simulink model "drone_model"  (R2020b)
settings: Solver=FixedStepAuto  StartTime=0.0  StopTime=30  FixedStep=0.01  RelTol=1e-3
undefined symbols (not defined in the file or in its folder): cd, clientID, d, g, I, Kf, Km, m, rho, sendCoppelia, sim
libraries: pid_lib x6, vrlib x1
settings Model: Creator=roger  LastModifiedBy=Guillermo
settings DataIOCC: ReturnWorkspaceOutputs=off

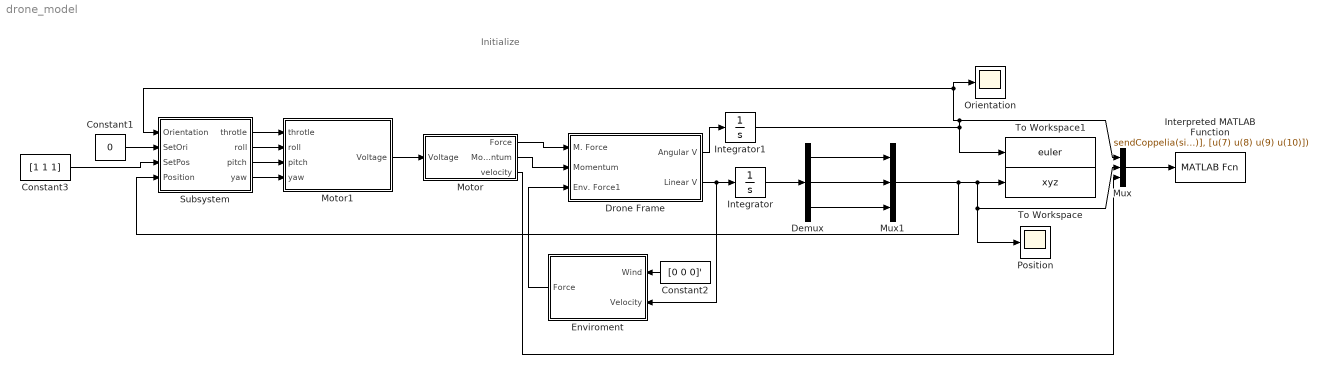
== system drone_model ==
  note: Initialize
  Constant1 : Constant  Value=0
  Constant2 : Constant  Value=[0 0 0]'  VectorParams1D=off
  Constant3 : Constant  Value=[1 1 1]
  Demux : Demux  Outputs=3
  Drone Frame : Subsystem
  Enviroment : Subsystem
  Integrator : Integrator
  Integrator1 : Integrator
  Interpreted MATLAB Function : MATLABFcn  MATLABFcn=sendCoppelia(sim, clientID, [u(4) u(5) u(6)], [u(1) u(2) u(3)], [u(7) u(8) u(9) u(10)])  OutputDimensions=0
  Motor : Subsystem
  Motor1 : Subsystem
  Mux : Mux  Inputs=3
  Mux1 : Mux  Inputs=3
  Orientation : Scope
  Position : Scope
  Subsystem : Subsystem
  To Workspace : ToWorkspace  VariableName=xyz  SaveFormat=Timeseries  SampleTime=-1
  To Workspace1 : ToWorkspace  VariableName=euler  SaveFormat=Timeseries  SampleTime=-1
  wires:
  Drone Frame/2(Linear V) -> Enviroment/2(Velocity), Integrator/1
  Drone Frame/1(Angular V) -> Integrator1/1
  Integrator1/1 -> To Workspace1/1, Mux/1, Subsystem/1(Orientation), Orientation/1
  Motor/1(Force) -> Drone Frame/1(M. Force)
  Motor/2(Momentum) -> Drone Frame/2(Momentum)
  Enviroment/1(Force) -> Drone Frame/3(Env. Force1)
  Constant2/1 -> Enviroment/1(Wind)
  Motor1/1(Voltage) -> Motor/1(Voltage)
  Integrator/1 -> Demux/1
  Subsystem/1(throtle) -> Motor1/1(throtle)
  Subsystem/2(roll) -> Motor1/2(roll)
  Subsystem/3(pitch) -> Motor1/3(pitch)
  Constant3/1 -> Subsystem/3(SetPos)
  Constant1/1 -> Subsystem/2(SetOri)
  Mux/1 -> Interpreted MATLAB Function/1
  Subsystem/4(yaw) -> Motor1/4(yaw)
  Mux1/1 -> Subsystem/4(Position), To Workspace/1, Mux/2, Position/1
  Demux/1 -> Mux1/1
  Demux/2 -> Mux1/2
  Demux/3 -> Mux1/3
  Motor/3(velocity) -> Mux/3

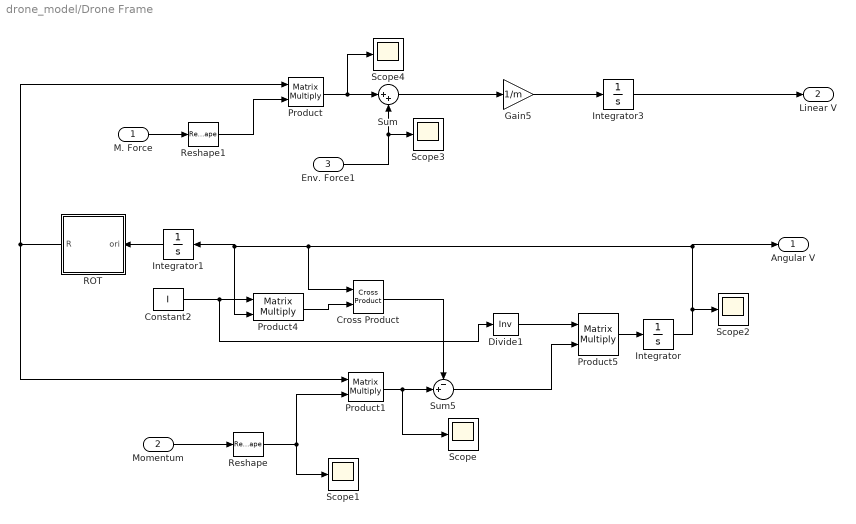
== system drone_model/Drone Frame ==
  M. Force : Inport
  Momentum : Inport  Port=2
  Env. Force1 : Inport  Port=3
  Constant2 : Constant  Value=I
  Cross Product : vrlib/Utilities/Cross Product
  Divide1 : Product  Inputs=/  Multiplication=Matrix(*)
  Gain5 : Gain  Gain=1/m
  Integrator : Integrator
  Integrator1 : Integrator
  Integrator3 : Integrator
  Product{,1,4..5} (4 alike) : Product  Multiplication=Matrix(*)
  ROT : MATLAB Function  TreatAsAtomicUnit=on
  Reshape : Reshape  OutputDimensionality=Column vector (2-D)
  Reshape1 : Reshape  OutputDimensionality=Column vector (2-D)
  Scope{,1..4} (5 alike) : Scope
  Sum : Sum  Inputs=|++
  Sum5 : Sum  Inputs=-+|
  Angular V : Outport
  Linear V : Outport  Port=2
  wires:
  Product/1 -> Scope4/1, Sum/1
  Sum5/1 -> Product5/2
  Gain5/1 -> Integrator3/1
  Sum/1 -> Gain5/1
  Product5/1 -> Integrator/1
  Integrator/1 -> Scope2/1, Integrator1/1, Product4/2, Cross Product/1, Angular V/1
  Cross Product/1 -> Sum5/1
  Divide1/1 -> Product5/1
  Constant2/1 -> Divide1/1, Product4/1
  Product4/1 -> Cross Product/2
  Integrator3/1 -> Linear V/1
  Momentum/1 -> Reshape/1
  M. Force/1 -> Reshape1/1
  Reshape1/1 -> Product/2
  Reshape/1 -> Scope1/1, Product1/2
  Product1/1 -> Scope/1, Sum5/2
  Env. Force1/1 -> Scope3/1, Sum/2
  Integrator1/1 -> ROT/1(ori)
  ROT/1(R) -> Product1/1, Product/1

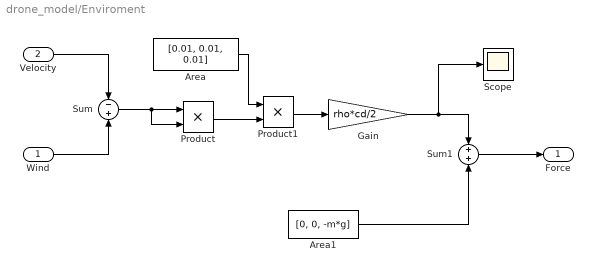
== system drone_model/Enviroment ==
  Wind : Inport
  Velocity : Inport  Port=2
  Area : Constant  Value=[0.01, 0.01, 0.01]
  Area1 : Constant  Value=[0, 0, -m*g]
  Gain : Gain  Gain=rho*cd/2
  Product : Product
  Product1 : Product
  Scope : Scope
  Sum : Sum  Inputs=-|+
  Sum1 : Sum  Inputs=+|+
  Force : Outport
  wires:
  Wind/1 -> Sum/2
  Velocity/1 -> Sum/1
  Sum/1 -> Product/2, Product/1
  Product/1 -> Product1/2
  Area/1 -> Product1/1
  Sum1/1 -> Force/1
  Area1/1 -> Sum1/2
  Product1/1 -> Gain/1
  Gain/1 -> Scope/1, Sum1/1

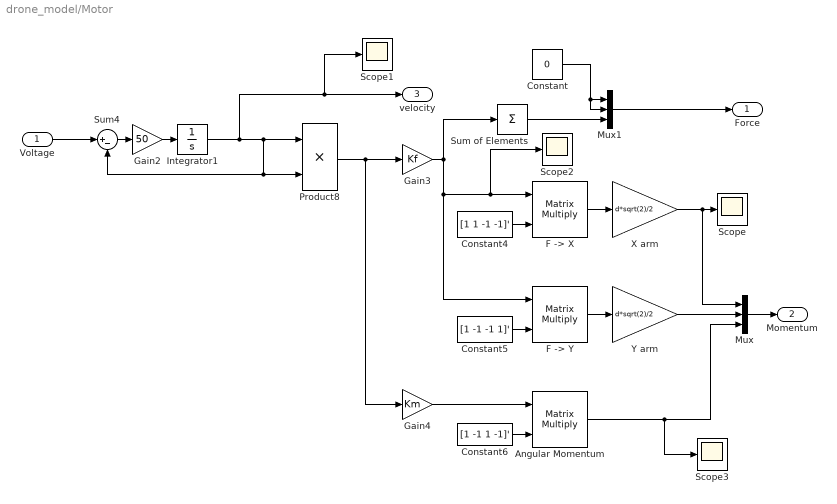
== system drone_model/Motor ==
  Voltage : Inport
  Angular Momentum : Product  Multiplication=Matrix(*)
  Constant : Constant  Value=0
  Constant4 : Constant  Value=[1 1 -1 -1]'  VectorParams1D=off
  Constant5 : Constant  Value=[1 -1 -1 1]'  VectorParams1D=off
  Constant6 : Constant  Value=[1 -1 1 -1]'  VectorParams1D=off
  "F -> X" : Product  Multiplication=Matrix(*)
  "F -> Y" : Product  Multiplication=Matrix(*)
  Gain2 : Gain  Gain=50
  Gain3 : Gain  Gain=Kf
  Gain4 : Gain  Gain=Km
  Integrator1 : Integrator
  Mux : Mux  Inputs=3
  Mux1 : Mux  Inputs=3
  Product8 : Product
  Scope{,1..3} (4 alike) : Scope
  Sum of Elements : Sum  Inputs=+
  Sum4 : Sum  Inputs=|+-
  X arm : Gain  Gain=d*sqrt(2)/2
  Y arm : Gain  Gain=d*sqrt(2)/2
  Force : Outport
  Momentum : Outport  Port=2
  velocity : Outport  Port=3
  wires:
  Gain3/1 -> Scope2/1, "F -> X"/1, "F -> Y"/1, Sum of Elements/1
  Sum4/1 -> Gain2/1
  Gain4/1 -> Angular Momentum/1
  Product8/1 -> Gain3/1, Gain4/1
  Integrator1/1 -> Scope1/1, velocity/1, Product8/1, Product8/2, Sum4/2
  "F -> Y"/1 -> Y arm/1
  Gain2/1 -> Integrator1/1
  Constant4/1 -> "F -> X"/2
  Constant6/1 -> Angular Momentum/2
  Constant5/1 -> "F -> Y"/2
  Voltage/1 -> Sum4/1
  "F -> X"/1 -> X arm/1
  X arm/1 -> Scope/1, Mux/1
  Y arm/1 -> Mux/2
  Angular Momentum/1 -> Scope3/1, Mux/3
  Mux/1 -> Momentum/1
  Sum of Elements/1 -> Mux1/3
  Mux1/1 -> Force/1
  Constant/1 -> Mux1/2, Mux1/1

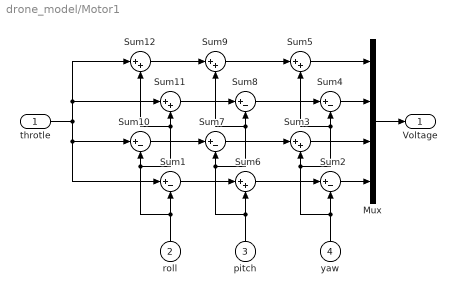
== system drone_model/Motor1 ==
  throtle : Inport
  roll : Inport  Port=2
  pitch : Inport  Port=3
  yaw : Inport  Port=4
  Mux : Mux
  Sum{1..2,4,7..8,10} (6 alike) : Sum  Inputs=|+-
  Sum{3,5..6,9,11..12} (6 alike) : Sum  Inputs=|++
  Voltage : Outport
  wires:
  Mux/1 -> Voltage/1
  Sum2/1 -> Mux/4
  yaw/1 -> Sum3/2, Sum5/2, Sum4/2, Sum2/2
  Sum3/1 -> Mux/3
  Sum4/1 -> Mux/2
  Sum5/1 -> Mux/1
  Sum8/1 -> Sum4/1
  Sum6/1 -> Sum2/1
  Sum9/1 -> Sum5/1
  Sum7/1 -> Sum3/1
  pitch/1 -> Sum7/2, Sum9/2, Sum8/2, Sum6/2
  throtle/1 -> Sum10/1, Sum1/1, Sum12/1, Sum11/1
  Sum11/1 -> Sum8/1
  Sum1/1 -> Sum6/1
  Sum12/1 -> Sum9/1
  Sum10/1 -> Sum7/1
  roll/1 -> Sum10/2, Sum12/2, Sum11/2, Sum1/2

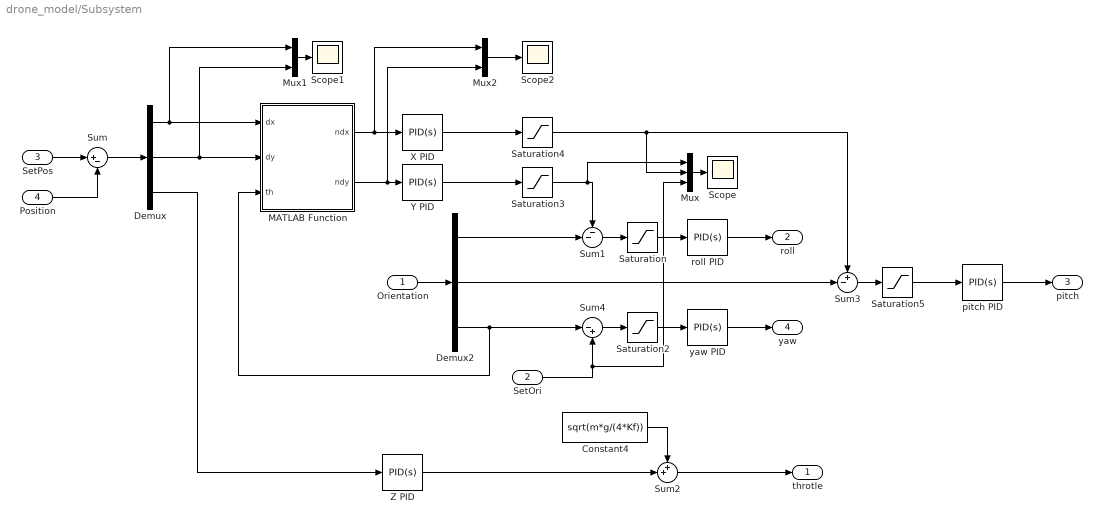
== system drone_model/Subsystem ==
  Orientation : Inport
  SetOri : Inport  Port=2
  SetPos : Inport  Port=3
  Position : Inport  Port=4
  Constant4 : Constant  Value=sqrt(m*g/(4*Kf))
  Demux : Demux  Outputs=3
  Demux2 : Demux  Outputs=3
  MATLAB Function : MATLAB Function  TreatAsAtomicUnit=on
  Mux : Mux  Inputs=3
  Mux1 : Mux  Inputs=2
  Mux2 : Mux  Inputs=2
  Saturation : Saturate  UpperLimit=0.01  LowerLimit=-0.01
  Saturation2 : Saturate  UpperLimit=0.01  LowerLimit=-0.01
  Saturation3 : Saturate  UpperLimit=0.05  LowerLimit=-0.05
  Saturation4 : Saturate  UpperLimit=0.05  LowerLimit=-0.05
  Saturation5 : Saturate  UpperLimit=0.01  LowerLimit=-0.01
  Scope : Scope
  Scope1 : Scope
  Scope2 : Scope
  Sum : Sum  Inputs=|+-
  Sum1 : Sum  Inputs=--|
  Sum2 : Sum  Inputs=++|
  Sum3 : Sum  Inputs=+-|
  Sum4 : Sum  Inputs=|-+
  X PID : pid_lib/PID Controller  Controller=PID  Form=Parallel  TimeDomain=Continuous-time  UseExternalTs=off  SampleTime=-1  IntegratorMethod=Forward Euler  FilterMethod=Forward Euler  ControllerParametersSource=internal  P=0.1  I=0  D=0.2  UseFilter=on  N=100  TunerSelectOption=Transfer Function Based (PID Tuner App)  InitialConditionSource=internal  InitialConditionForIntegrator=0  InitialConditionForFilter=0  DifferentiatorICPrevScaledInput=0  ExternalReset=none  TrackingMode=off  Kt=1  LimitOutput=off  SatLimitsSource=internal  UpperSaturationLimit=inf  LowerSaturationLimit=-inf  LinearizeAsGain=on  AntiWindupMode=none  Kb=1  POutMin=[]  POutMax=[]  IOutMin=[]  IOutMax=[]  DOutMin=[]  DOutMax=[]  NOutMin=[]  NOutMax=[]  SumOutMin=[]  SumOutMax=[]  SaturationOutMin=[]  SaturationOutMax=[]  PParamMin=[]  PParamMax=[]  IParamMin=[]  IParamMax=[]  DParamMin=[]  DParamMax=[]  NParamMin=[]  NParamMax=[]  KbParamMin=[]  KbParamMax=[]  KtParamMin=[]  KtParamMax=[]  KbOutMin=[]  KbOutMax=[]  KtOutMin=[]  KtOutMax=[]  IntegratorOutMin=[]  IntegratorOutMax=[]  FilterOutMin=[]  FilterOutMax=[]  SumI1OutMin=[]  SumI1OutMax=[]  SumI2OutMin=[]  SumI2OutMax=[]  SumI3OutMin=[]  SumI3OutMax=[]  SumI4OutMin=[]  SumI4OutMax=[]  SumDOutMin=[]  SumDOutMax=[]  DifferentiatorOutMin=[]  DifferentiatorOutMax=[]  FilterDiffOutCoefMin=[]  FilterDiffOutCoefMax=[]  ReciprocalOutMin=[]  ReciprocalOutMax=[]  SumDenOutMin=[]  SumDenOutMax=[]  SumNumOutMin=[]  SumNumOutMax=[]  DivideOutMin=[]  DivideOutMax=[]  UdiffTsProdOutMin=[]  UdiffTsProdOutMax=[]  NTsProdOutMin=[]  NTsProdOutMax=[]  UintegralTsProdOutMin=[]  UintegralTsProdOutMax=[]  UngainTsProdOutMin=[]  UngainTsProdOutMax=[]  IntegratorContinuousStateAttributes=''  IntegratorStateMustResolveToSignalObject=off  IntegratorRTWStateStorageClass=Auto  FilterContinuousStateAttributes=''  FilterStateMustResolveToSignalObject=off  FilterRTWStateStorageClass=Auto  ParallelPVariant=InternalParameters  IdealPVariant=Disabled  IVariant=InternalParameters  DVariant=InternalParameters  IntegratorVariant=Continuous  SatVariant=Disabled  AWVariant=Passthrough  PCopyVariant=Disabled  TRVariant=Disabled  FdbkBlocksVariant=Forward  IdealPFdbkVariant=Disabled  SatFdbkVariant=Disabled  DerivativeFilterVariant=ContFilter  NVariant=InternalParameters  NCopyVariant=Disabled  FilterICVariant=InternalICsFilter  IntegratorICVariant=InternalICs  ExternalResetVariant=Disabled  TRSumVariant=Passthrough  SumFdbkVariant=Disabled  SumVariant=Sum_PID  TsampFilterVariant=InternalTs  TsampNgainVariant=Passthrough  TsampIntegralVariant=Passthrough  ExternalSaturationOutDataTypeStr=Inherit: Same as second input
  Y PID : pid_lib/PID Controller  Controller=PID  Form=Parallel  TimeDomain=Continuous-time  UseExternalTs=off  SampleTime=-1  IntegratorMethod=Forward Euler  FilterMethod=Forward Euler  ControllerParametersSource=internal  P=0.1  I=0  D=0.2  UseFilter=on  N=100  TunerSelectOption=Transfer Function Based (PID Tuner App)  InitialConditionSource=internal  InitialConditionForIntegrator=0  InitialConditionForFilter=0  DifferentiatorICPrevScaledInput=0  ExternalReset=none  TrackingMode=off  Kt=1  LimitOutput=off  SatLimitsSource=internal  UpperSaturationLimit=inf  LowerSaturationLimit=-inf  LinearizeAsGain=on  AntiWindupMode=none  Kb=1  POutMin=[]  POutMax=[]  IOutMin=[]  IOutMax=[]  DOutMin=[]  DOutMax=[]  NOutMin=[]  NOutMax=[]  SumOutMin=[]  SumOutMax=[]  SaturationOutMin=[]  SaturationOutMax=[]  PParamMin=[]  PParamMax=[]  IParamMin=[]  IParamMax=[]  DParamMin=[]  DParamMax=[]  NParamMin=[]  NParamMax=[]  KbParamMin=[]  KbParamMax=[]  KtParamMin=[]  KtParamMax=[]  KbOutMin=[]  KbOutMax=[]  KtOutMin=[]  KtOutMax=[]  IntegratorOutMin=[]  IntegratorOutMax=[]  FilterOutMin=[]  FilterOutMax=[]  SumI1OutMin=[]  SumI1OutMax=[]  SumI2OutMin=[]  SumI2OutMax=[]  SumI3OutMin=[]  SumI3OutMax=[]  SumI4OutMin=[]  SumI4OutMax=[]  SumDOutMin=[]  SumDOutMax=[]  DifferentiatorOutMin=[]  DifferentiatorOutMax=[]  FilterDiffOutCoefMin=[]  FilterDiffOutCoefMax=[]  ReciprocalOutMin=[]  ReciprocalOutMax=[]  SumDenOutMin=[]  SumDenOutMax=[]  SumNumOutMin=[]  SumNumOutMax=[]  DivideOutMin=[]  DivideOutMax=[]  UdiffTsProdOutMin=[]  UdiffTsProdOutMax=[]  NTsProdOutMin=[]  NTsProdOutMax=[]  UintegralTsProdOutMin=[]  UintegralTsProdOutMax=[]  UngainTsProdOutMin=[]  UngainTsProdOutMax=[]  IntegratorContinuousStateAttributes=''  IntegratorStateMustResolveToSignalObject=off  IntegratorRTWStateStorageClass=Auto  FilterContinuousStateAttributes=''  FilterStateMustResolveToSignalObject=off  FilterRTWStateStorageClass=Auto  ParallelPVariant=InternalParameters  IdealPVariant=Disabled  IVariant=InternalParameters  DVariant=InternalParameters  IntegratorVariant=Continuous  SatVariant=Disabled  AWVariant=Passthrough  PCopyVariant=Disabled  TRVariant=Disabled  FdbkBlocksVariant=Forward  IdealPFdbkVariant=Disabled  SatFdbkVariant=Disabled  DerivativeFilterVariant=ContFilter  NVariant=InternalParameters  NCopyVariant=Disabled  FilterICVariant=InternalICsFilter  IntegratorICVariant=InternalICs  ExternalResetVariant=Disabled  TRSumVariant=Passthrough  SumFdbkVariant=Disabled  SumVariant=Sum_PID  TsampFilterVariant=InternalTs  TsampNgainVariant=Passthrough  TsampIntegralVariant=Passthrough  ExternalSaturationOutDataTypeStr=Inherit: Same as second input
  Z PID : pid_lib/PID Controller  Controller=PID  Form=Parallel  TimeDomain=Continuous-time  UseExternalTs=off  SampleTime=-1  IntegratorMethod=Forward Euler  FilterMethod=Forward Euler  ControllerParametersSource=internal  P=0.05  I=0  D=0.2  UseFilter=on  N=100  TunerSelectOption=Transfer Function Based (PID Tuner App)  InitialConditionSource=internal  InitialConditionForIntegrator=0  InitialConditionForFilter=0  DifferentiatorICPrevScaledInput=0  ExternalReset=none  TrackingMode=off  Kt=1  LimitOutput=off  SatLimitsSource=internal  UpperSaturationLimit=inf  LowerSaturationLimit=-inf  LinearizeAsGain=on  AntiWindupMode=none  Kb=1  POutMin=[]  POutMax=[]  IOutMin=[]  IOutMax=[]  DOutMin=[]  DOutMax=[]  NOutMin=[]  NOutMax=[]  SumOutMin=[]  SumOutMax=[]  SaturationOutMin=[]  SaturationOutMax=[]  PParamMin=[]  PParamMax=[]  IParamMin=[]  IParamMax=[]  DParamMin=[]  DParamMax=[]  NParamMin=[]  NParamMax=[]  KbParamMin=[]  KbParamMax=[]  KtParamMin=[]  KtParamMax=[]  KbOutMin=[]  KbOutMax=[]  KtOutMin=[]  KtOutMax=[]  IntegratorOutMin=[]  IntegratorOutMax=[]  FilterOutMin=[]  FilterOutMax=[]  SumI1OutMin=[]  SumI1OutMax=[]  SumI2OutMin=[]  SumI2OutMax=[]  SumI3OutMin=[]  SumI3OutMax=[]  SumI4OutMin=[]  SumI4OutMax=[]  SumDOutMin=[]  SumDOutMax=[]  DifferentiatorOutMin=[]  DifferentiatorOutMax=[]  FilterDiffOutCoefMin=[]  FilterDiffOutCoefMax=[]  ReciprocalOutMin=[]  ReciprocalOutMax=[]  SumDenOutMin=[]  SumDenOutMax=[]  SumNumOutMin=[]  SumNumOutMax=[]  DivideOutMin=[]  DivideOutMax=[]  UdiffTsProdOutMin=[]  UdiffTsProdOutMax=[]  NTsProdOutMin=[]  NTsProdOutMax=[]  UintegralTsProdOutMin=[]  UintegralTsProdOutMax=[]  UngainTsProdOutMin=[]  UngainTsProdOutMax=[]  IntegratorContinuousStateAttributes=''  IntegratorStateMustResolveToSignalObject=off  IntegratorRTWStateStorageClass=Auto  FilterContinuousStateAttributes=''  FilterStateMustResolveToSignalObject=off  FilterRTWStateStorageClass=Auto  ParallelPVariant=InternalParameters  IdealPVariant=Disabled  IVariant=InternalParameters  DVariant=InternalParameters  IntegratorVariant=Continuous  SatVariant=Disabled  AWVariant=Passthrough  PCopyVariant=Disabled  TRVariant=Disabled  FdbkBlocksVariant=Forward  IdealPFdbkVariant=Disabled  SatFdbkVariant=Disabled  DerivativeFilterVariant=ContFilter  NVariant=InternalParameters  NCopyVariant=Disabled  FilterICVariant=InternalICsFilter  IntegratorICVariant=InternalICs  ExternalResetVariant=Disabled  TRSumVariant=Passthrough  SumFdbkVariant=Disabled  SumVariant=Sum_PID  TsampFilterVariant=InternalTs  TsampNgainVariant=Passthrough  TsampIntegralVariant=Passthrough  ExternalSaturationOutDataTypeStr=Inherit: Same as second input
  pitch PID : pid_lib/PID Controller  Controller=PID  Form=Parallel  TimeDomain=Continuous-time  UseExternalTs=off  SampleTime=-1  IntegratorMethod=Forward Euler  FilterMethod=Forward Euler  ControllerParametersSource=internal  P=0.1  I=0  D=0.2  UseFilter=on  N=100  TunerSelectOption=Transfer Function Based (PID Tuner App)  InitialConditionSource=internal  InitialConditionForIntegrator=0  InitialConditionForFilter=0  DifferentiatorICPrevScaledInput=0  ExternalReset=none  TrackingMode=off  Kt=1  LimitOutput=off  SatLimitsSource=internal  UpperSaturationLimit=inf  LowerSaturationLimit=-inf  LinearizeAsGain=on  AntiWindupMode=none  Kb=1  POutMin=[]  POutMax=[]  IOutMin=[]  IOutMax=[]  DOutMin=[]  DOutMax=[]  NOutMin=[]  NOutMax=[]  SumOutMin=[]  SumOutMax=[]  SaturationOutMin=[]  SaturationOutMax=[]  PParamMin=[]  PParamMax=[]  IParamMin=[]  IParamMax=[]  DParamMin=[]  DParamMax=[]  NParamMin=[]  NParamMax=[]  KbParamMin=[]  KbParamMax=[]  KtParamMin=[]  KtParamMax=[]  KbOutMin=[]  KbOutMax=[]  KtOutMin=[]  KtOutMax=[]  IntegratorOutMin=[]  IntegratorOutMax=[]  FilterOutMin=[]  FilterOutMax=[]  SumI1OutMin=[]  SumI1OutMax=[]  SumI2OutMin=[]  SumI2OutMax=[]  SumI3OutMin=[]  SumI3OutMax=[]  SumI4OutMin=[]  SumI4OutMax=[]  SumDOutMin=[]  SumDOutMax=[]  DifferentiatorOutMin=[]  DifferentiatorOutMax=[]  FilterDiffOutCoefMin=[]  FilterDiffOutCoefMax=[]  ReciprocalOutMin=[]  ReciprocalOutMax=[]  SumDenOutMin=[]  SumDenOutMax=[]  SumNumOutMin=[]  SumNumOutMax=[]  DivideOutMin=[]  DivideOutMax=[]  UdiffTsProdOutMin=[]  UdiffTsProdOutMax=[]  NTsProdOutMin=[]  NTsProdOutMax=[]  UintegralTsProdOutMin=[]  UintegralTsProdOutMax=[]  UngainTsProdOutMin=[]  UngainTsProdOutMax=[]  IntegratorContinuousStateAttributes=''  IntegratorStateMustResolveToSignalObject=off  IntegratorRTWStateStorageClass=Auto  FilterContinuousStateAttributes=''  FilterStateMustResolveToSignalObject=off  FilterRTWStateStorageClass=Auto  ParallelPVariant=InternalParameters  IdealPVariant=Disabled  IVariant=InternalParameters  DVariant=InternalParameters  IntegratorVariant=Continuous  SatVariant=Disabled  AWVariant=Passthrough  PCopyVariant=Disabled  TRVariant=Disabled  FdbkBlocksVariant=Forward  IdealPFdbkVariant=Disabled  SatFdbkVariant=Disabled  DerivativeFilterVariant=ContFilter  NVariant=InternalParameters  NCopyVariant=Disabled  FilterICVariant=InternalICsFilter  IntegratorICVariant=InternalICs  ExternalResetVariant=Disabled  TRSumVariant=Passthrough  SumFdbkVariant=Disabled  SumVariant=Sum_PID  TsampFilterVariant=InternalTs  TsampNgainVariant=Passthrough  TsampIntegralVariant=Passthrough  ExternalSaturationOutDataTypeStr=Inherit: Same as second input
  roll PID : pid_lib/PID Controller  Controller=PID  Form=Parallel  TimeDomain=Continuous-time  UseExternalTs=off  SampleTime=-1  IntegratorMethod=Forward Euler  FilterMethod=Forward Euler  ControllerParametersSource=internal  P=0.1  I=0  D=0.2  UseFilter=on  N=100  TunerSelectOption=Transfer Function Based (PID Tuner App)  InitialConditionSource=internal  InitialConditionForIntegrator=0  InitialConditionForFilter=0  DifferentiatorICPrevScaledInput=0  ExternalReset=none  TrackingMode=off  Kt=1  LimitOutput=off  SatLimitsSource=internal  UpperSaturationLimit=inf  LowerSaturationLimit=-inf  LinearizeAsGain=on  AntiWindupMode=none  Kb=1  POutMin=[]  POutMax=[]  IOutMin=[]  IOutMax=[]  DOutMin=[]  DOutMax=[]  NOutMin=[]  NOutMax=[]  SumOutMin=[]  SumOutMax=[]  SaturationOutMin=[]  SaturationOutMax=[]  PParamMin=[]  PParamMax=[]  IParamMin=[]  IParamMax=[]  DParamMin=[]  DParamMax=[]  NParamMin=[]  NParamMax=[]  KbParamMin=[]  KbParamMax=[]  KtParamMin=[]  KtParamMax=[]  KbOutMin=[]  KbOutMax=[]  KtOutMin=[]  KtOutMax=[]  IntegratorOutMin=[]  IntegratorOutMax=[]  FilterOutMin=[]  FilterOutMax=[]  SumI1OutMin=[]  SumI1OutMax=[]  SumI2OutMin=[]  SumI2OutMax=[]  SumI3OutMin=[]  SumI3OutMax=[]  SumI4OutMin=[]  SumI4OutMax=[]  SumDOutMin=[]  SumDOutMax=[]  DifferentiatorOutMin=[]  DifferentiatorOutMax=[]  FilterDiffOutCoefMin=[]  FilterDiffOutCoefMax=[]  ReciprocalOutMin=[]  ReciprocalOutMax=[]  SumDenOutMin=[]  SumDenOutMax=[]  SumNumOutMin=[]  SumNumOutMax=[]  DivideOutMin=[]  DivideOutMax=[]  UdiffTsProdOutMin=[]  UdiffTsProdOutMax=[]  NTsProdOutMin=[]  NTsProdOutMax=[]  UintegralTsProdOutMin=[]  UintegralTsProdOutMax=[]  UngainTsProdOutMin=[]  UngainTsProdOutMax=[]  IntegratorContinuousStateAttributes=''  IntegratorStateMustResolveToSignalObject=off  IntegratorRTWStateStorageClass=Auto  FilterContinuousStateAttributes=''  FilterStateMustResolveToSignalObject=off  FilterRTWStateStorageClass=Auto  ParallelPVariant=InternalParameters  IdealPVariant=Disabled  IVariant=InternalParameters  DVariant=InternalParameters  IntegratorVariant=Continuous  SatVariant=Disabled  AWVariant=Passthrough  PCopyVariant=Disabled  TRVariant=Disabled  FdbkBlocksVariant=Forward  IdealPFdbkVariant=Disabled  SatFdbkVariant=Disabled  DerivativeFilterVariant=ContFilter  NVariant=InternalParameters  NCopyVariant=Disabled  FilterICVariant=InternalICsFilter  IntegratorICVariant=InternalICs  ExternalResetVariant=Disabled  TRSumVariant=Passthrough  SumFdbkVariant=Disabled  SumVariant=Sum_PID  TsampFilterVariant=InternalTs  TsampNgainVariant=Passthrough  TsampIntegralVariant=Passthrough  ExternalSaturationOutDataTypeStr=Inherit: Same as second input
  yaw PID : pid_lib/PID Controller  Controller=PID  Form=Parallel  TimeDomain=Continuous-time  UseExternalTs=off  SampleTime=-1  IntegratorMethod=Forward Euler  FilterMethod=Forward Euler  ControllerParametersSource=internal  P=0.01  I=0  D=0.03  UseFilter=on  N=100  TunerSelectOption=Transfer Function Based (PID Tuner App)  InitialConditionSource=internal  InitialConditionForIntegrator=0  InitialConditionForFilter=0  DifferentiatorICPrevScaledInput=0  ExternalReset=none  TrackingMode=off  Kt=1  LimitOutput=off  SatLimitsSource=internal  UpperSaturationLimit=inf  LowerSaturationLimit=-inf  LinearizeAsGain=on  AntiWindupMode=none  Kb=1  POutMin=[]  POutMax=[]  IOutMin=[]  IOutMax=[]  DOutMin=[]  DOutMax=[]  NOutMin=[]  NOutMax=[]  SumOutMin=[]  SumOutMax=[]  SaturationOutMin=[]  SaturationOutMax=[]  PParamMin=[]  PParamMax=[]  IParamMin=[]  IParamMax=[]  DParamMin=[]  DParamMax=[]  NParamMin=[]  NParamMax=[]  KbParamMin=[]  KbParamMax=[]  KtParamMin=[]  KtParamMax=[]  KbOutMin=[]  KbOutMax=[]  KtOutMin=[]  KtOutMax=[]  IntegratorOutMin=[]  IntegratorOutMax=[]  FilterOutMin=[]  FilterOutMax=[]  SumI1OutMin=[]  SumI1OutMax=[]  SumI2OutMin=[]  SumI2OutMax=[]  SumI3OutMin=[]  SumI3OutMax=[]  SumI4OutMin=[]  SumI4OutMax=[]  SumDOutMin=[]  SumDOutMax=[]  DifferentiatorOutMin=[]  DifferentiatorOutMax=[]  FilterDiffOutCoefMin=[]  FilterDiffOutCoefMax=[]  ReciprocalOutMin=[]  ReciprocalOutMax=[]  SumDenOutMin=[]  SumDenOutMax=[]  SumNumOutMin=[]  SumNumOutMax=[]  DivideOutMin=[]  DivideOutMax=[]  UdiffTsProdOutMin=[]  UdiffTsProdOutMax=[]  NTsProdOutMin=[]  NTsProdOutMax=[]  UintegralTsProdOutMin=[]  UintegralTsProdOutMax=[]  UngainTsProdOutMin=[]  UngainTsProdOutMax=[]  IntegratorContinuousStateAttributes=''  IntegratorStateMustResolveToSignalObject=off  IntegratorRTWStateStorageClass=Auto  FilterContinuousStateAttributes=''  FilterStateMustResolveToSignalObject=off  FilterRTWStateStorageClass=Auto  ParallelPVariant=InternalParameters  IdealPVariant=Disabled  IVariant=InternalParameters  DVariant=InternalParameters  IntegratorVariant=Continuous  SatVariant=Disabled  AWVariant=Passthrough  PCopyVariant=Disabled  TRVariant=Disabled  FdbkBlocksVariant=Forward  IdealPFdbkVariant=Disabled  SatFdbkVariant=Disabled  DerivativeFilterVariant=ContFilter  NVariant=InternalParameters  NCopyVariant=Disabled  FilterICVariant=InternalICsFilter  IntegratorICVariant=InternalICs  ExternalResetVariant=Disabled  TRSumVariant=Passthrough  SumFdbkVariant=Disabled  SumVariant=Sum_PID  TsampFilterVariant=InternalTs  TsampNgainVariant=Passthrough  TsampIntegralVariant=Passthrough  ExternalSaturationOutDataTypeStr=Inherit: Same as second input
  throtle : Outport
  roll : Outport  Port=2
  pitch : Outport  Port=3
  yaw : Outport  Port=4
  wires:
  Sum2/1 -> throtle/1
  Z PID/1 -> Sum2/2
  Position/1 -> Sum/2
  Constant4/1 -> Sum2/1
  SetPos/1 -> Sum/1
  Sum/1 -> Demux/1
  Demux/1 -> Mux1/1, MATLAB Function/1(dx)
  X PID/1 -> Saturation4/1
  Y PID/1 -> Saturation3/1
  Orientation/1 -> Demux2/1
  SetOri/1 -> Mux/3, Sum4/2
  Sum3/1 -> Saturation5/1
  Demux2/3 -> MATLAB Function/3(th), Sum4/1
  roll PID/1 -> roll/1
  Saturation4/1 -> Mux/2, Sum3/1
  Sum1/1 -> Saturation/1
  Demux2/1 -> Sum1/2
  Saturation2/1 -> yaw PID/1
  yaw PID/1 -> yaw/1
  Demux2/2 -> Sum3/2
  Sum4/1 -> Saturation2/1
  Saturation/1 -> roll PID/1
  pitch PID/1 -> pitch/1
  Saturation3/1 -> Mux/1, Sum1/1
  Demux/2 -> Mux1/2, MATLAB Function/2(dy)
  Mux/1 -> Scope/1
  Mux1/1 -> Scope1/1
  Mux2/1 -> Scope2/1
  MATLAB Function/2(ndy) -> Mux2/2, Y PID/1
  MATLAB Function/1(ndx) -> Mux2/1, X PID/1
  Saturation5/1 -> pitch PID/1
  Demux/3 -> Z PID/1

== matlab function drone_model/Drone Frame/ROT ==
  data: ori input; R output
function R = rot(ori)
    roll = ori(1); pitch = ori(2) ; yaw = ori(3);
    R = [ cos(pitch)*cos(yaw) - sin(pitch)*sin(roll)*sin(yaw), -cos(roll)*sin(yaw), cos(yaw)*sin(pitch) + cos(pitch)*sin(roll)*sin(yaw); ...
          cos(pitch)*sin(yaw) + cos(yaw)*sin(pitch)*sin(roll),  cos(roll)*cos(yaw), sin(pitch)*sin(yaw) - cos(pitch)*cos(yaw)*sin(roll); ...
                                        -cos(roll)*sin(pitch),           sin(roll),                                cos(pitch)*cos(roll)];
end

== matlab function drone_model/Subsystem/MATLAB Function ==
  data: dx input; ndx output; dy input; ndy output; th input
function [ndx,ndy] = rotate(dx, dy, th)
  alpha = atan2(dy,dx);
  r = sqrt(dx*dx+ dy*dy);
  ndx = r*cos(alpha-th);
  ndy = r*sin(alpha-th);
end
